simulink model "SeatSensingLeft"  (R2015a)
settings: Solver=FixedStepDiscrete  StartTime=0.0  StopTime=10.0  FixedStep=0.1  RelTol=1e-3
settings Model: Creator=Morya  LastModifiedBy=Morya
settings DataIOCC: SaveFormat=StructureWithTime
settings OptimizationCC: ZeroExternalMemoryAtStartup=off  ZeroInternalMemoryAtStartup=off  OptimizeModelRefInitCode=on  LifeSpan=1.0
settings ModelReferenceCC: ModelReferenceNumInstancesAllowed=Single
settings RTWCC: SystemTargetFile=autosar.tlc  GenCodeOnly=on  TemplateMakefile=ert_default_tmf  Description=AUTOSAR
settings CodeAppCC: IgnoreCustomStorageClasses=off
settings STFCustomTargetCC: GenerateSampleERTMain=off  ParMdlRefBuildCompliant=on  CompOptLevelCompliant=on  IncludeMdlTerminateFcn=off  CombineOutputUpdateFcns=on  SuppressErrorStatus=on  ERTFirstTimeCompliant=on  SupportNonFinite=off  SupportComplex=off  SupportContinuousTime=off  SupportVariableSizeSignals=off  AutosarCompliant=on  SystemTargetFile=autosar.tlc
settings ERTTargetCC: GenerateSampleERTMain=off  ParMdlRefBuildCompliant=on  CompOptLevelCompliant=on  IncludeMdlTerminateFcn=off  SuppressErrorStatus=on  ERTFirstTimeCompliant=on  SupportNonFinite=off  SupportComplex=off  SupportContinuousTime=off  SupportVariableSizeSignals=off  AutosarCompliant=on  ERTCustomFileTemplate=example_file_process.tlc

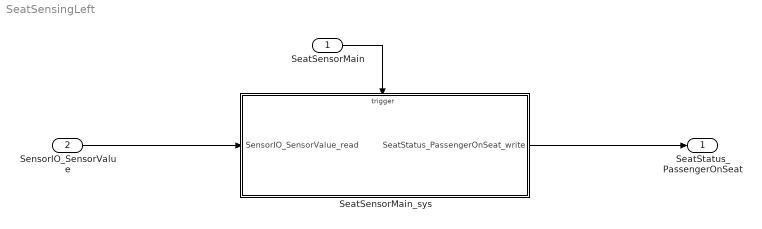
== system SeatSensingLeft ==
  SeatSensorMain : Inport  OutputFunctionCall=on
  SensorIO_SensorValue : Inport  Port=2  OutDataTypeStr=boolean  PortDimensions=1
  SeatSensorMain_sys : Subsystem
  SeatStatus_PassengerOnSeat : Outport  OutDataTypeStr=boolean  PortDimensions=1
  wires:
  SeatSensorMain/1 -> SeatSensorMain_sys/Trigger
  SensorIO_SensorValue/1 -> SeatSensorMain_sys/1(SensorIO_SensorValue_read)
  SeatSensorMain_sys/1(SeatStatus_PassengerOnSeat_write) -> SeatStatus_PassengerOnSeat/1

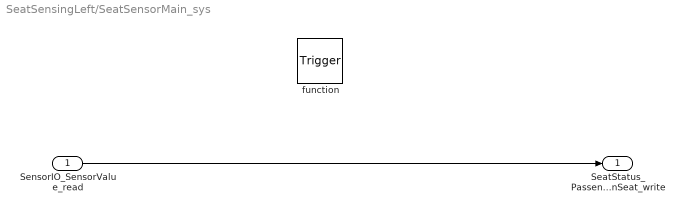
== system SeatSensingLeft/SeatSensorMain_sys ==
  SensorIO_SensorValue_read : Inport
  function : TriggerPort  TriggerType=function-call
  SeatStatus_PassengerOnSeat_write : Outport
  wires:
  SensorIO_SensorValue_read/1 -> SeatStatus_PassengerOnSeat_write/1
